simulink model "missile_model_3"  (R2022b)
settings: Solver=ode4  StartTime=0.0  StopTime=50  FixedStep=0.01  RelTol=1e-3
InitFcn:
  | clc, clear, close all
  | UAV_Data
  | Sim_Parameters
values from neighbouring files (symbols this model uses):
  Alt_Trim = 0    [Missile_Trim_Solution.mat]    (also in Trim_Main_missile.m = 4000; Trim_Solution_missile1.mat; Trim_Solution_missile2.mat; Trim_Solution_missile3.mat)
  D = 0.150    (= 0.15)    [UAV_Data.m]    (also in UAV_Data.mat)
  G_Turn = Turn_dot_Trim * Speed_Trim / UNIT_GRAV    [Trim_Main_missile.m]
  Gamma_Trim = 0.0 * UNIT_DEG2RAD    [Trim_Main_missile.m]
  Init_Cnstr1 = 0.0    (= 0)    [Trim_Main_missile.m]
  Init_Cnstr2 = 0.0    (= 0)    [Trim_Main_missile.m]
  Init_Cnstr3 = 0.0    (= 0)    [Trim_Main_missile.m]
  K_A = 0.0270    (= 0.027)    [UAV_Data.m]    (also in UAV_Data.mat)
  K_DC = 0.8443/10    (= 0.08443)    [UAV_Data.m]    (also in UAV_Data.mat = 0.8443)
  K_p = 0.01    [UAV_Data.m]    (also in UAV_Data.mat)
  K_phi = 20.0*2    (= 40)    [UAV_Data.m]    (also in UAV_Data.mat = 20)
  K_R = 0.0777    [UAV_Data.m]    (also in UAV_Data.mat)
  Mass = 30.0    (= 30)    [UAV_Data.m]    (also in UAV_Data.mat)
  Omega_i = -6.5208/5    (= -1.30416)    [UAV_Data.m]    (also in UAV_Data.mat = -6.5208)
  S = dat.S    [Assigment3_work.m]    (also in Missile_EoM.m; UAV_Data.m = 0.0176714586764; UAV_Data.mat = 0.0176714586764; verify_coeff.m)
  Speed_Trim = 102.088237307    [Missile_Trim_Solution.mat]    (also in Trim_Main_missile.m = 227.1878; Trim_Solution_missile1.mat = 102.0804; Trim_Solution_missile2.mat = 136.1072; Trim_Solution_missile3.mat = 204.1608)
  UNIT_GRAV = 9.81    [Sim_Parameters.m]
  Wn_Act = 25.0 * 2 * pi    (= 157.079632679)    [UAV_Data.m]    (also in UAV_Data.mat)
  Zeta_Act = 0.707    [UAV_Data.m]    (also in UAV_Data.mat)
libraries: aerolibconvert2 x3, aerolibasang x2, shared6dof x1, aerolibtransform2 x1, aerolibatmos2 x1
settings Model: Creator=Komsun  LastModifiedBy=Komsun

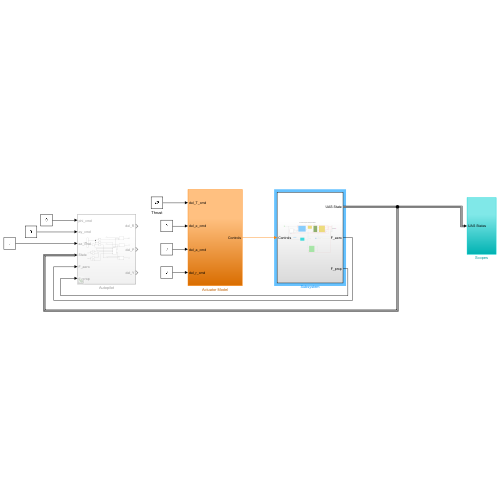
[thumbnail: Simulink's stored preview of the top-level diagram]
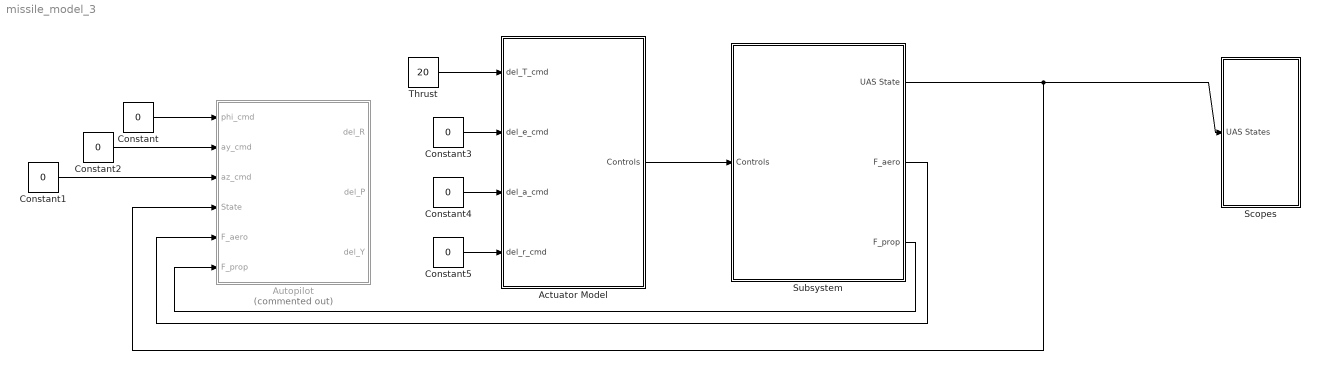
== system missile_model_3 ==
  Actuator Model : Subsystem
  Autopilot : Subsystem  Commented=on
  Constant{,1..5} (6 alike) : Constant  Value=0
  Scopes : Subsystem
  Subsystem : Subsystem
  Thrust : Constant  Value=20
  wires:
  Subsystem/1(UAS State) -> Autopilot/4(State), Scopes/1(UAS States)
  Constant/1 -> Autopilot/1(phi_cmd)
  Thrust/1 -> Actuator Model/1(del_T_cmd)
  Constant1/1 -> Autopilot/3(az_cmd)
  Actuator Model/1(Controls) -> Subsystem/1(Controls)
  Constant2/1 -> Autopilot/2(ay_cmd)
  Subsystem/2(F_aero) -> Autopilot/5(F_aero)
  Subsystem/3(F_prop) -> Autopilot/6(F_prop)
  Constant3/1 -> Actuator Model/2(del_e_cmd)
  Constant4/1 -> Actuator Model/3(del_a_cmd)
  Constant5/1 -> Actuator Model/4(del_r_cmd)

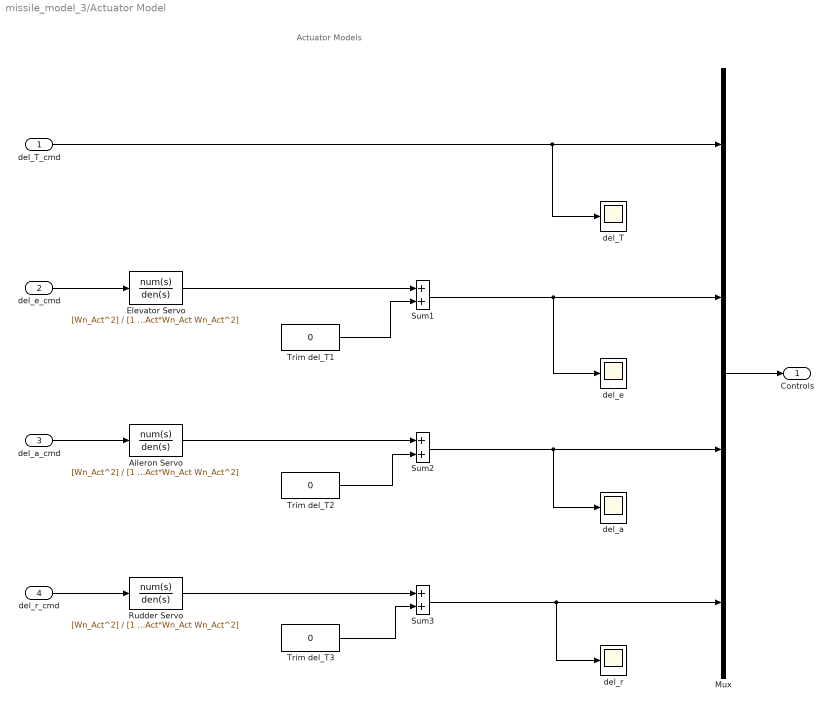
== system missile_model_3/Actuator Model ==
  note: Actuator Models
  del_T_cmd : Inport
  del_e_cmd : Inport  Port=2
  del_a_cmd : Inport  Port=3
  del_r_cmd : Inport  Port=4
  Aileron Servo : TransferFcn  Numerator=[Wn_Act^2]  Denominator=[1 2*Zeta_Act*Wn_Act Wn_Act^2]
  Elevator Servo : TransferFcn  Numerator=[Wn_Act^2]  Denominator=[1 2*Zeta_Act*Wn_Act Wn_Act^2]
  Mux : Mux
  Rudder Servo : TransferFcn  Numerator=[Wn_Act^2]  Denominator=[1 2*Zeta_Act*Wn_Act Wn_Act^2]
  Sum1 : Sum  SaturateOnIntegerOverflow=on
  Sum2 : Sum  SaturateOnIntegerOverflow=on
  Sum3 : Sum  SaturateOnIntegerOverflow=on
  Trim del_T1 : Constant  Value=0
  Trim del_T2 : Constant  Value=0
  Trim del_T3 : Constant  Value=0
  del_T : Scope
  del_a : Scope
  del_e : Scope
  del_r : Scope
  Controls : Outport
  wires:
  Mux/1 -> Controls/1
  del_T_cmd/1 -> del_T/1, Mux/1
  del_e_cmd/1 -> Elevator Servo/1
  Elevator Servo/1 -> Sum1/1
  Sum1/1 -> del_e/1, Mux/2
  Trim del_T1/1 -> Sum1/2
  Sum2/1 -> del_a/1, Mux/3
  Aileron Servo/1 -> Sum2/1
  Trim del_T2/1 -> Sum2/2
  del_a_cmd/1 -> Aileron Servo/1
  Sum3/1 -> del_r/1, Mux/4
  Trim del_T3/1 -> Sum3/2
  Rudder Servo/1 -> Sum3/1
  del_r_cmd/1 -> Rudder Servo/1

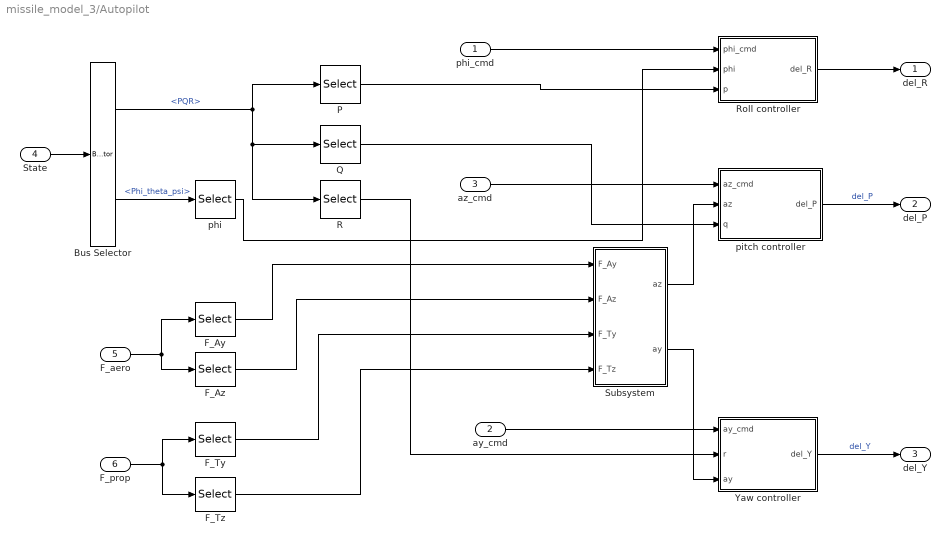
== system missile_model_3/Autopilot ==
  phi_cmd : Inport
  ay_cmd : Inport  Port=2
  az_cmd : Inport  Port=3
  State : Inport  Port=4
  F_aero : Inport  Port=5
  F_prop : Inport  Port=6
  Bus Selector : BusSelector  OutputSignals=PQR,Phi_theta_psi
  F_Ay : Selector  InputPortWidth=3  IndexOptions=Index vector (dialog)  Indices=[2]  OutputSizes=1
  F_Az : Selector  InputPortWidth=3  IndexOptions=Index vector (dialog)  Indices=[3]  OutputSizes=1
  F_Ty : Selector  InputPortWidth=3  IndexOptions=Index vector (dialog)  Indices=[2]  OutputSizes=1
  F_Tz : Selector  InputPortWidth=3  IndexOptions=Index vector (dialog)  Indices=[3]  OutputSizes=1
  P : Selector  InputPortWidth=3  IndexOptions=Index vector (dialog)  Indices=[1]  OutputSizes=1
  Q : Selector  InputPortWidth=3  IndexOptions=Index vector (dialog)  Indices=[2]  OutputSizes=1
  R : Selector  InputPortWidth=3  IndexOptions=Index vector (dialog)  Indices=[3]  OutputSizes=1
  Roll controller : Subsystem
  Subsystem : Subsystem
  Yaw controller : Subsystem
  phi : Selector  InputPortWidth=3  IndexOptions=Index vector (dialog)  Indices=[1]  OutputSizes=1
  pitch controller : Subsystem
  del_R : Outport
  del_P : Outport  Port=2
  del_Y : Outport  Port=3
  wires:
  pitch controller/1(del_P) -> del_P/1  "del_P"
  Yaw controller/1(del_Y) -> del_Y/1  "del_Y"
  phi_cmd/1 -> Roll controller/1(phi_cmd)
  Roll controller/1(del_R) -> del_R/1
  az_cmd/1 -> pitch controller/1(az_cmd)
  Subsystem/1(az) -> pitch controller/2(az)
  ay_cmd/1 -> Yaw controller/1(ay_cmd)
  Subsystem/2(ay) -> Yaw controller/3(ay)
  State/1 -> Bus Selector/1
  F_aero/1 -> F_Az/1, F_Ay/1
  F_Ay/1 -> Subsystem/1(F_Ay)
  F_Az/1 -> Subsystem/2(F_Az)
  F_prop/1 -> F_Ty/1, F_Tz/1
  F_Ty/1 -> Subsystem/3(F_Ty)
  F_Tz/1 -> Subsystem/4(F_Tz)
  Bus Selector/1 -> R/1, Q/1, P/1  "<PQR>"
  P/1 -> Roll controller/3(p)
  Q/1 -> pitch controller/3(q)
  R/1 -> Yaw controller/2(r)
  Bus Selector/2 -> phi/1  "<Phi_theta_psi>"
  phi/1 -> Roll controller/2(phi)

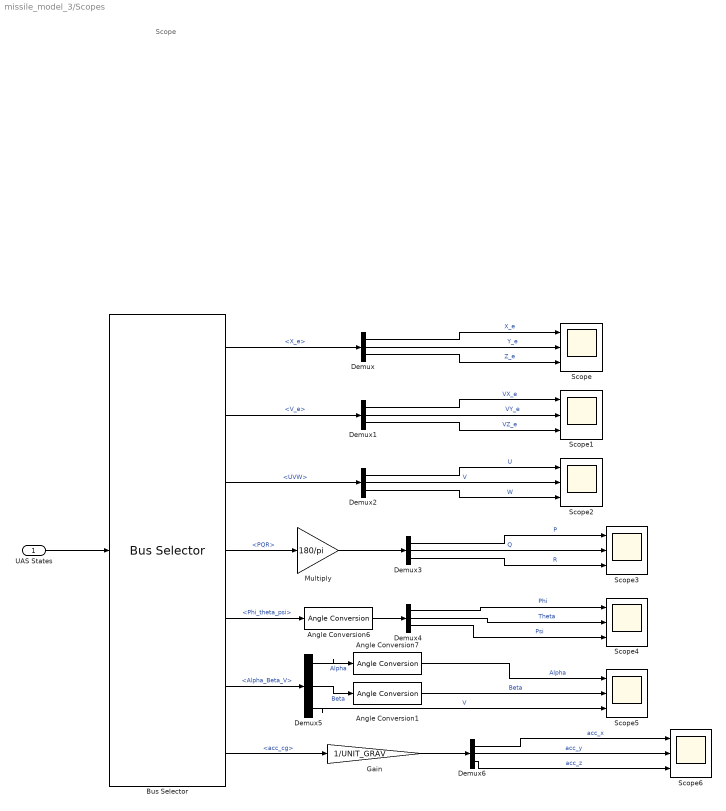
== system missile_model_3/Scopes ==
  note: Scope
  UAS States : Inport
  Angle Conversion1 : aerolibconvert2/Angle Conversion  IU=rad  OU=deg
  Angle Conversion6 : aerolibconvert2/Angle Conversion  IU=rad  OU=deg
  Angle Conversion7 : aerolibconvert2/Angle Conversion  IU=rad  OU=deg
  Bus Selector : BusSelector  OutputSignals=X_e,V_e,UVW,PQR,Phi_theta_psi,Alpha_Beta_V,acc_cg
  Demux{,1..6} (7 alike) : Demux  Outputs=3
  Gain : Gain  Gain=1/UNIT_GRAV
  Multiply : Gain  Gain=180/pi
  Scope{,1..6} (7 alike) : Scope  NumInputPorts=3
  wires:
  UAS States/1 -> Bus Selector/1
  Demux/1 -> Scope/1  "X_e"
  Demux/2 -> Scope/2  "Y_e"
  Demux/3 -> Scope/3  "Z_e"
  Bus Selector/4 -> Multiply/1  "<PQR>"
  Bus Selector/5 -> Angle Conversion6/1  "<Phi_theta_psi>"
  Bus Selector/6 -> Demux5/1  "<Alpha_Beta_V>"
  Bus Selector/7 -> Gain/1  "<acc_cg>"
  Bus Selector/1 -> Demux/1  "<X_e>"
  Demux1/3 -> Scope1/3  "VZ_e"
  Demux1/1 -> Scope1/1  "VX_e"
  Demux1/2 -> Scope1/2  "VY_e"
  Bus Selector/2 -> Demux1/1  "<V_e>"
  Bus Selector/3 -> Demux2/1  "<UVW>"
  Demux2/2 -> Scope2/2  "V"
  Demux2/1 -> Scope2/1  "U"
  Demux2/3 -> Scope2/3  "W"
  Demux3/3 -> Scope3/3  "R"
  Demux3/1 -> Scope3/1  "P"
  Demux3/2 -> Scope3/2  "Q"
  Multiply/1 -> Demux3/1
  Angle Conversion6/1 -> Demux4/1
  Demux4/2 -> Scope4/2  "Theta"
  Demux4/1 -> Scope4/1  "Phi"
  Demux4/3 -> Scope4/3  "Psi"
  Demux5/2 -> Angle Conversion1/1  "Beta"
  Demux5/3 -> Scope5/3  "V"
  Demux5/1 -> Angle Conversion7/1  "Alpha"
  Demux6/1 -> Scope6/1  "acc_x"
  Demux6/2 -> Scope6/2  "acc_y"
  Gain/1 -> Demux6/1
  Demux6/3 -> Scope6/3  "acc_z"
  Angle Conversion7/1 -> Scope5/1  "Alpha"
  Angle Conversion1/1 -> Scope5/2  "Beta"

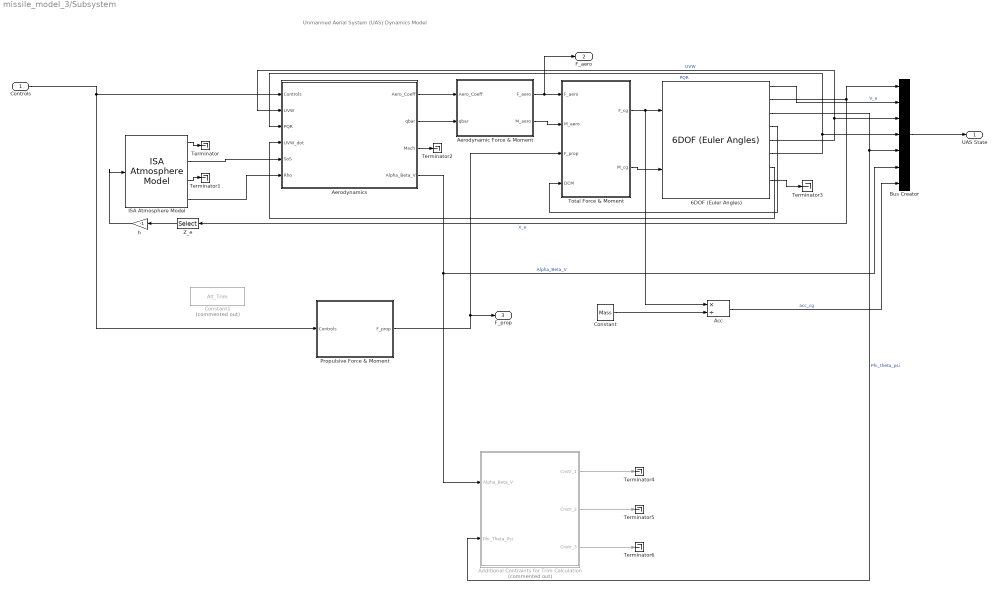
== system missile_model_3/Subsystem ==
  note: Unmanned Aerial System (UAS) Dynamics Model
  Controls : Inport
  6DOF (Euler Angles) : shared6dof/6DOF (Euler Angles)  units=Metric (MKS)  mtype=Fixed  rep=Euler Angles  xme_0=Init_Pos  Vm_0=Init_Vel  eul_0=[0 0 0]  pm_0=[0 0 0]  mass_0=30  mass_e=0.5  mass_f=2.0  inertia=I_TENSOR  inertia_e=eye(3)  inertia_f=2*eye(3)  k_quat=1.0  vre_flag=on  abi_flag=on  aMode=0  xme_statename=''  Vm_statename=''  eul_statename=''  quat_statename=''  pm_statename=''  mass_statename=''
  Acc : Product  Inputs=*/  RndMeth=Zero
  Additional Contraints for Trim Calculation : Subsystem  Commented=on
  Aerodynamic Force & Moment : Subsystem
  Aerodynamics : Subsystem
  Bus Creator : BusCreator  Inputs=7
  Constant : Constant  Value=Mass
  Constant1 : Constant  Commented=on  Value=Alt_Trim
  ISA Atmosphere Model : aerolibatmos2/ISA Atmosphere Model  custom=off  g=9.80665  gamma=1.4  R=287.0531  L=0.0065  h_trop=11000  h_strat=20000  rho0=1.225  P0=101325  T0=288.15  h0=0
  Propulsive Force & Moment : Subsystem
  Terminator{,1..6} (7 alike) : Terminator
  Total Force & Moment : Subsystem
  Z_e : Selector  InputPortWidth=3  IndexOptions=Index vector (dialog)  Indices=[3]  OutputSizes=1
  h : Gain  Gain=-1
  UAS State : Outport
  F_aero : Outport  Port=2
  F_prop : Outport  Port=3
  wires:
  6DOF (Euler Angles)/3 -> Bus Creator/5, Additional Contraints for Trim Calculation/2(Phi_Theta_Psi)  "Phi_theta_psi"
  Additional Contraints for Trim Calculation/2(Cnstr_2) -> Terminator5/1
  Aerodynamics/4(Alpha_Beta_V) -> Bus Creator/6, Additional Contraints for Trim Calculation/1(Alpha_Beta_V)  "Alpha_Beta_V"
  Propulsive Force & Moment/1(F_prop) -> F_prop/1, Total Force & Moment/3(F_prop)
  Additional Contraints for Trim Calculation/1(Cnstr_1) -> Terminator4/1
  h/1 -> ISA Atmosphere Model/1
  ISA Atmosphere Model/2 -> Aerodynamics/5(SoS)
  6DOF (Euler Angles)/7 -> Aerodynamics/4("UVW_dot ")
  Z_e/1 -> h/1
  Aerodynamics/1(Aero_Coeff) -> Aerodynamic Force & Moment/1(Aero_Coeff)
  Aerodynamic Force & Moment/1(F_aero) -> F_aero/1, Total Force & Moment/1(F_aero)
  ISA Atmosphere Model/1 -> Terminator/1
  ISA Atmosphere Model/3 -> Terminator1/1
  Acc/1 -> Bus Creator/7  "acc_cg"
  6DOF (Euler Angles)/5 -> Bus Creator/3, Aerodynamics/2(UVW)  "UVW"
  Controls/1 -> Propulsive Force & Moment/1(Controls), Aerodynamics/1(Controls)
  Aerodynamic Force & Moment/2(M_aero) -> Total Force & Moment/2(M_aero)
  Aerodynamics/3(Mach) -> Terminator2/1
  Aerodynamics/2(qbar) -> Aerodynamic Force & Moment/2(qbar)
  Additional Contraints for Trim Calculation/3(Cnstr_3) -> Terminator6/1
  Total Force & Moment/1(F_cg) -> Acc/1, 6DOF (Euler Angles)/1
  Total Force & Moment/2(M_cg) -> 6DOF (Euler Angles)/2
  6DOF (Euler Angles)/1 -> Bus Creator/2  "V_e"
  Constant/1 -> Acc/2
  ISA Atmosphere Model/4 -> Aerodynamics/6(Rho)
  6DOF (Euler Angles)/6 -> Bus Creator/4, Aerodynamics/3(PQR)  "PQR"
  6DOF (Euler Angles)/2 -> Z_e/1, Bus Creator/1  "X_e"
  6DOF (Euler Angles)/4 -> Total Force & Moment/4(DCM)
  Bus Creator/1 -> UAS State/1
  6DOF (Euler Angles)/8 -> Terminator3/1

== system missile_model_3/Autopilot/Roll controller ==
  phi_cmd : Inport
  phi : Inport  Port=2
  p : Inport  Port=3
  K_p : Gain  Gain=K_p
  K_phi : Gain  Gain=K_phi
  Sum : Sum  Inputs=|+-
  Sum1 : Sum  Inputs=|+-
  del_R : Outport
  wires:
  p/1 -> Sum/2
  K_p/1 -> del_R/1  "del_R"
  Sum/1 -> K_phi/1
  phi/1 -> Sum1/2
  Sum1/1 -> K_p/1
  K_phi/1 -> Sum1/1
  phi_cmd/1 -> Sum/1

== system missile_model_3/Autopilot/Subsystem ==
  F_Ay : Inport
  F_Az : Inport  Port=2
  F_Ty : Inport  Port=3
  F_Tz : Inport  Port=4
  Divide : Product  Inputs=*/
  Divide1 : Product  Inputs=*/
  Mass : Constant  Value=Mass
  Sum : Sum  Inputs=|++
  Sum1 : Sum  Inputs=|++
  az : Outport
  ay : Outport  Port=2
  wires:
  F_Ay/1 -> Sum1/1  "F_Ay"
  Mass/1 -> Divide1/2, Divide/2
  Sum/1 -> Divide/1
  F_Ty/1 -> Sum1/2  "F_Ty"
  Sum1/1 -> Divide1/1
  F_Az/1 -> Sum/1  "F_Az"
  Divide/1 -> az/1
  F_Tz/1 -> Sum/2  "F_Tz"
  Divide1/1 -> ay/1

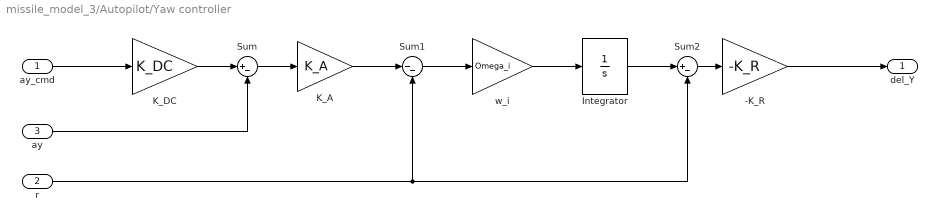
== system missile_model_3/Autopilot/Yaw controller ==
  ay_cmd : Inport
  r : Inport  Port=2
  ay : Inport  Port=3
  -K_R : Gain  Gain=-K_R
  Integrator : Integrator
  K_A : Gain  Gain=K_A
  K_DC : Gain  Gain=K_DC
  Sum : Sum  Inputs=|+-
  Sum1 : Sum  Inputs=|--
  Sum2 : Sum  Inputs=|+-
  w_i : Gain  Gain=Omega_i
  del_Y : Outport
  wires:
  ay_cmd/1 -> K_DC/1
  r/1 -> Sum2/2, Sum1/2
  K_DC/1 -> Sum/1
  ay/1 -> Sum/2
  Sum/1 -> K_A/1
  K_A/1 -> Sum1/1
  Sum1/1 -> w_i/1
  w_i/1 -> Integrator/1
  Integrator/1 -> Sum2/1
  Sum2/1 -> -K_R/1
  -K_R/1 -> del_Y/1

== system missile_model_3/Autopilot/pitch controller ==
  az_cmd : Inport
  az : Inport  Port=2
  q : Inport  Port=3
  Integrator : Integrator
  K_A : Gain  Gain=K_A
  K_DC : Gain  Gain=K_DC
  K_R : Gain  Gain=K_R
  Sum : Sum  Inputs=|+-
  Sum1 : Sum  Inputs=|-+
  Sum2 : Sum  Inputs=|++
  w_i : Gain  Gain=Omega_i
  del_P : Outport
  wires:
  az_cmd/1 -> K_DC/1
  K_DC/1 -> Sum/1
  az/1 -> Sum/2
  Sum/1 -> K_A/1
  K_A/1 -> Sum1/1
  q/1 -> Sum2/2, Sum1/2
  Sum1/1 -> w_i/1
  w_i/1 -> Integrator/1
  Integrator/1 -> Sum2/1
  Sum2/1 -> K_R/1
  K_R/1 -> del_P/1

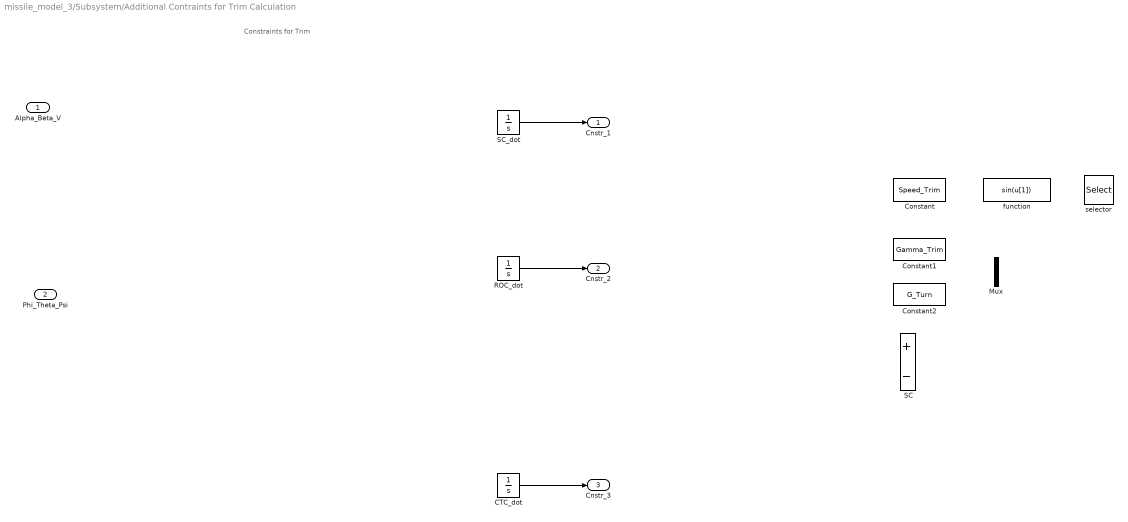
== system missile_model_3/Subsystem/Additional Contraints for Trim Calculation ==
  note: Constraints for Trim
  Alpha_Beta_V : Inport  PortDimensions=3
  Phi_Theta_Psi : Inport  Port=2  PortDimensions=3
  CTC_dot : Integrator  InitialCondition=Init_Cnstr3
  Constant : Constant  Value=Speed_Trim
  Constant1 : Constant  Value=Gamma_Trim
  Constant2 : Constant  Value=G_Turn
  Mux : Mux  Inputs=2
  ROC_dot : Integrator  InitialCondition=Init_Cnstr2
  SC : Sum  Inputs=+-
  SC_dot : Integrator  InitialCondition=Init_Cnstr1
  function : Fcn
  selector : Selector  InputPortWidth=3  IndexOptions=Index vector (dialog)  Indices=[3]  OutputSizes=1
  Cnstr_1 : Outport
  Cnstr_2 : Outport  Port=2
  Cnstr_3 : Outport  Port=3
  wires:
  SC_dot/1 -> Cnstr_1/1
  ROC_dot/1 -> Cnstr_2/1
  CTC_dot/1 -> Cnstr_3/1

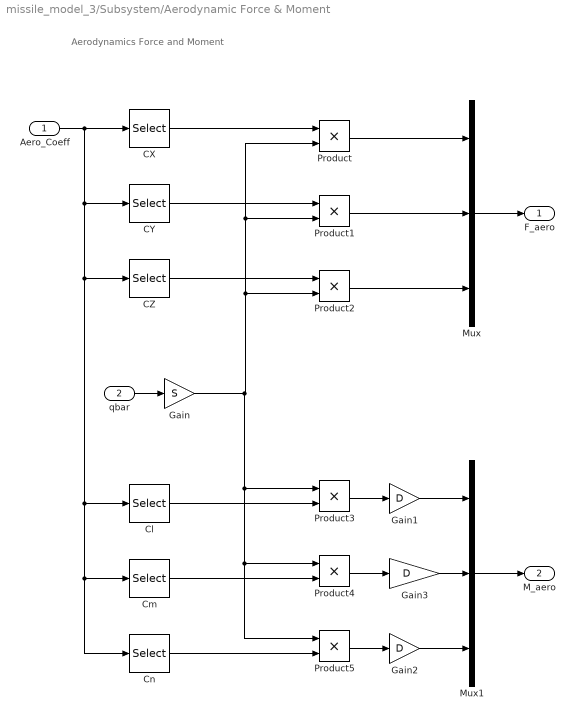
== system missile_model_3/Subsystem/Aerodynamic Force & Moment ==
  note: Aerodynamics Force and Moment
  Aero_Coeff : Inport
  qbar : Inport  Port=2
  CX : Selector  InputPortWidth=6  IndexOptions=Index vector (dialog)  Indices=[1]  OutputSizes=1
  CY : Selector  InputPortWidth=6  IndexOptions=Index vector (dialog)  Indices=[2]  OutputSizes=1
  CZ : Selector  InputPortWidth=6  IndexOptions=Index vector (dialog)  Indices=[3]  OutputSizes=1
  Cl : Selector  InputPortWidth=6  IndexOptions=Index vector (dialog)  Indices=[4]  OutputSizes=1
  Cm : Selector  InputPortWidth=6  IndexOptions=Index vector (dialog)  Indices=[5]  OutputSizes=1
  Cn : Selector  InputPortWidth=6  IndexOptions=Index vector (dialog)  Indices=[6]  OutputSizes=1
  Gain : Gain  Gain=S
  Gain1 : Gain  Gain=D
  Gain2 : Gain  Gain=D
  Gain3 : Gain  Gain=D
  Mux : Mux  Inputs=3
  Mux1 : Mux  Inputs=3
  Product{,1..5} (6 alike) : Product
  F_aero : Outport
  M_aero : Outport  Port=2
  wires:
  Aero_Coeff/1 -> Cl/1, Cn/1, Cm/1, CZ/1, CY/1, CX/1
  qbar/1 -> Gain/1
  CX/1 -> Product/1
  Gain/1 -> Product5/1, Product4/1, Product3/1, Product2/2, Product1/2, Product/2
  CY/1 -> Product1/1
  CZ/1 -> Product2/1
  Product/1 -> Mux/1
  Product1/1 -> Mux/2
  Product2/1 -> Mux/3
  Mux/1 -> F_aero/1
  Cl/1 -> Product3/2
  Cm/1 -> Product4/2
  Cn/1 -> Product5/2
  Product3/1 -> Gain1/1
  Product4/1 -> Gain3/1
  Product5/1 -> Gain2/1
  Mux1/1 -> M_aero/1
  Gain1/1 -> Mux1/1
  Gain2/1 -> Mux1/3
  Gain3/1 -> Mux1/2

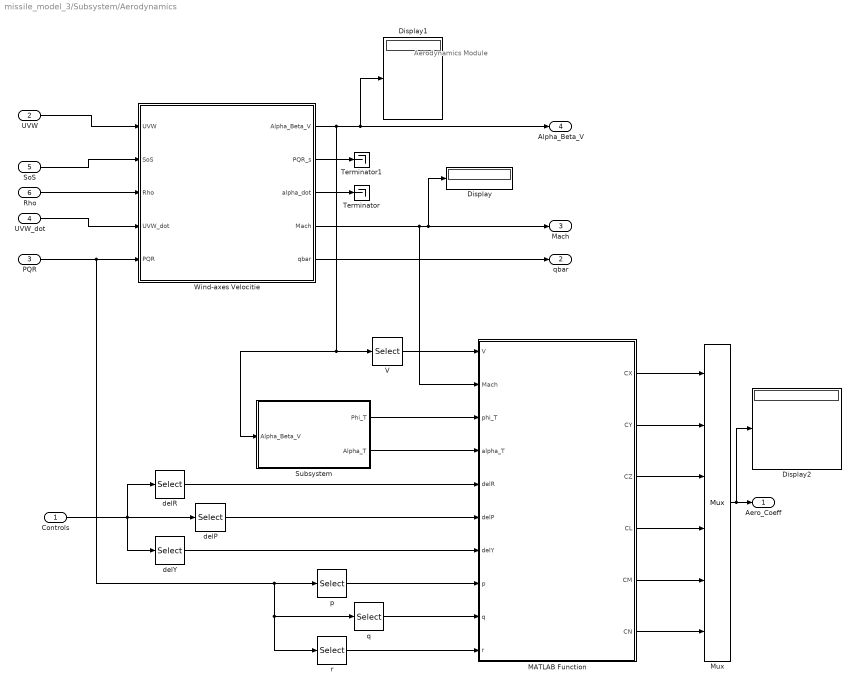
== system missile_model_3/Subsystem/Aerodynamics ==
  note: Aerodynamics Module
  Controls : Inport
  UVW : Inport  Port=2
  PQR : Inport  Port=3
  "UVW_dot " : Inport  Port=4
  SoS : Inport  Port=5
  Rho : Inport  Port=6
  Display : Display
  Display1 : Display
  Display2 : Display
  MATLAB Function : MATLAB Function  TreatAsAtomicUnit=on
  Mux : Mux  Inputs=6
  Subsystem : Subsystem
  Terminator : Terminator
  Terminator1 : Terminator
  V : Selector  InputPortWidth=3  IndexOptions=Index vector (dialog)  Indices=[3]  OutputSizes=1
  Wind-axes Velocitie : Subsystem
  delP : Selector  InputPortWidth=4  IndexOptions=Index vector (dialog)  Indices=[3]  OutputSizes=1
  delR : Selector  InputPortWidth=4  IndexOptions=Index vector (dialog)  Indices=[2]  OutputSizes=1
  delY : Selector  InputPortWidth=4  IndexOptions=Index vector (dialog)  Indices=[4]  OutputSizes=1
  p : Selector  InputPortWidth=3  IndexOptions=Index vector (dialog)  Indices=[1]  OutputSizes=1
  q : Selector  InputPortWidth=3  IndexOptions=Index vector (dialog)  Indices=[2]  OutputSizes=1
  r : Selector  InputPortWidth=3  IndexOptions=Index vector (dialog)  Indices=[3]  OutputSizes=1
  Aero_Coeff : Outport
  qbar : Outport  Port=2
  Mach : Outport  Port=3
  Alpha_Beta_V : Outport  Port=4
  wires:
  Wind-axes Velocitie/1(Alpha_Beta_V) -> Subsystem/1(Alpha_Beta_V), V/1, Display1/1, Alpha_Beta_V/1
  UVW/1 -> Wind-axes Velocitie/1(UVW)
  Mux/1 -> Display2/1, Aero_Coeff/1
  Wind-axes Velocitie/4(Mach) -> MATLAB Function/2(Mach), Mach/1, Display/1
  Wind-axes Velocitie/5(qbar) -> qbar/1
  SoS/1 -> Wind-axes Velocitie/2(SoS)
  Rho/1 -> Wind-axes Velocitie/3(Rho)
  "UVW_dot "/1 -> Wind-axes Velocitie/4(UVW_dot)
  PQR/1 -> r/1, q/1, p/1, Wind-axes Velocitie/5(PQR)
  Wind-axes Velocitie/3(alpha_dot) -> Terminator/1
  Wind-axes Velocitie/2(PQR_s) -> Terminator1/1
  Subsystem/2(Alpha_T) -> MATLAB Function/4(alpha_T)
  V/1 -> MATLAB Function/1(V)
  Subsystem/1(Phi_T) -> MATLAB Function/3(phi_T)
  Controls/1 -> delY/1, delR/1, delP/1
  delR/1 -> MATLAB Function/5(delR)
  delP/1 -> MATLAB Function/6(delP)
  delY/1 -> MATLAB Function/7(delY)
  p/1 -> MATLAB Function/8(p)
  q/1 -> MATLAB Function/9(q)
  r/1 -> MATLAB Function/10(r)
  MATLAB Function/1(CX) -> Mux/1
  MATLAB Function/2(CY) -> Mux/2
  MATLAB Function/3(CZ) -> Mux/3
  MATLAB Function/4(CL) -> Mux/4
  MATLAB Function/5(CM) -> Mux/5
  MATLAB Function/6(CN) -> Mux/6

== system missile_model_3/Subsystem/Propulsive Force & Moment ==
  note: Propulsive Force and Moment
  Controls : Inport
  Constant : Constant  Value=0
  Mux : Mux  Inputs=3
  Thrust : Selector  InputPortWidth=4  IndexOptions=Index vector (dialog)  Indices=[1]  OutputSizes=1
  F_prop : Outport
  wires:
  Constant/1 -> Mux/3, Mux/2
  Controls/1 -> Thrust/1
  Thrust/1 -> Mux/1
  Mux/1 -> F_prop/1

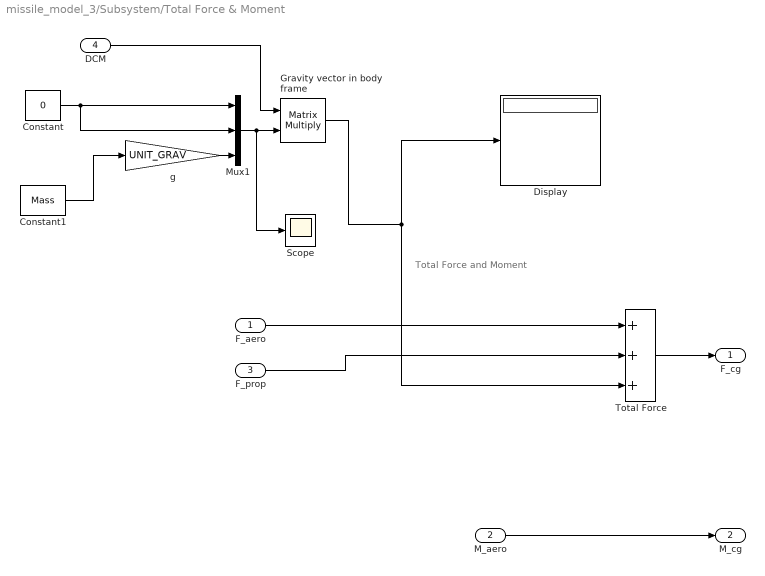
== system missile_model_3/Subsystem/Total Force & Moment ==
  note: Total Force and Moment
  F_aero : Inport  PortDimensions=3
  M_aero : Inport  Port=2  PortDimensions=3
  F_prop : Inport  Port=3  PortDimensions=3
  DCM : Inport  Port=4
  Constant : Constant  Value=0
  Constant1 : Constant  Value=Mass
  Display : Display
  "Gravity vector in body frame " : Product  Multiplication=Matrix(*)  InputSameDT=on  SaturateOnIntegerOverflow=on  OutDataTypeStr=Inherit: Same as first input
  Mux1 : Mux  Inputs=3
  Scope : Scope
  Total Force : Sum  Inputs=+++  InputSameDT=on  SaturateOnIntegerOverflow=on  OutDataTypeStr=Inherit: Same as first input
  g : Gain  Gain=UNIT_GRAV
  F_cg : Outport
  M_cg : Outport  Port=2
  wires:
  Total Force/1 -> F_cg/1
  F_aero/1 -> Total Force/1
  F_prop/1 -> Total Force/2
  M_aero/1 -> M_cg/1
  Mux1/1 -> Scope/1, "Gravity vector in body frame "/2
  "Gravity vector in body frame "/1 -> Total Force/3, Display/1
  Constant1/1 -> g/1
  Constant/1 -> Mux1/2, Mux1/1
  g/1 -> Mux1/3
  DCM/1 -> "Gravity vector in body frame "/1

== system missile_model_3/Subsystem/Aerodynamics/Subsystem ==
  Alpha_Beta_V : Inport
  Acos : Trigonometry  Operator=acos
  Atan2 : Trigonometry  Operator=atan2
  Beta : Selector  InputPortWidth=3  IndexOptions=Index vector (dialog)  Indices=[2]  OutputSizes=1
  Cos1 : Trigonometry  Operator=cos
  Cos2 : Trigonometry  Operator=cos
  Product : Product
  Sin : Trigonometry
  Tan : Trigonometry  Operator=tan
  alpha : Selector  InputPortWidth=3  IndexOptions=Index vector (dialog)  Indices=[1]  OutputSizes=1
  Phi_T : Outport
  Alpha_T : Outport  Port=2
  wires:
  Alpha_Beta_V/1 -> alpha/1, Beta/1
  Beta/1 -> Tan/1, Cos2/1
  Tan/1 -> Atan2/1
  Sin/1 -> Atan2/2
  Atan2/1 -> Phi_T/1
  alpha/1 -> Cos1/1, Sin/1
  Cos1/1 -> Product/1
  Cos2/1 -> Product/2
  Product/1 -> Acos/1
  Acos/1 -> Alpha_T/1

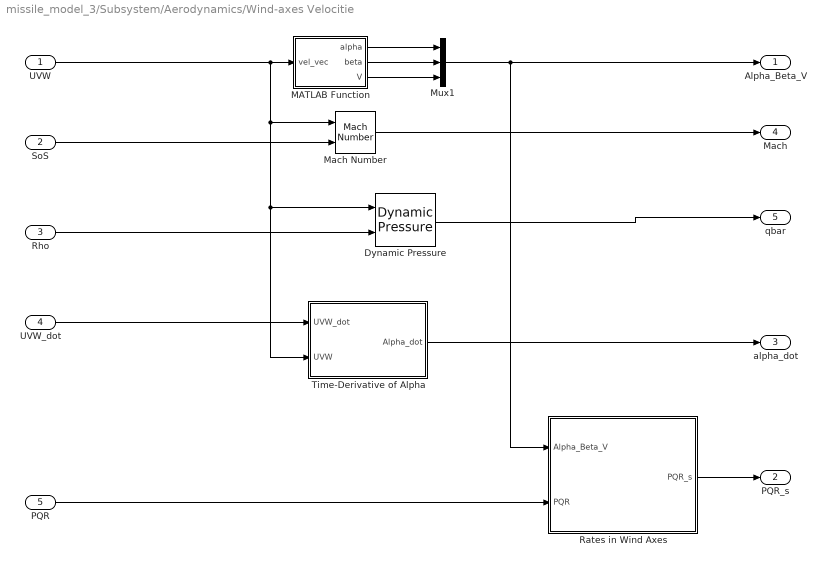
== system missile_model_3/Subsystem/Aerodynamics/Wind-axes Velocitie ==
  UVW : Inport
  SoS : Inport  Port=2
  Rho : Inport  Port=3
  UVW_dot : Inport  Port=4
  PQR : Inport  Port=5
  Dynamic Pressure : aerolibasang/Dynamic Pressure
  MATLAB Function : MATLAB Function  TreatAsAtomicUnit=on
  Mach Number : aerolibasang/Mach Number
  Mux1 : Mux  Inputs=3
  Rates in Wind Axes : Subsystem
  Time-Derivative of Alpha : Subsystem
  Alpha_Beta_V : Outport
  PQR_s : Outport  Port=2
  alpha_dot : Outport  Port=3
  Mach : Outport  Port=4
  qbar : Outport  Port=5
  wires:
  UVW_dot/1 -> Time-Derivative of Alpha/1(UVW_dot)
  Time-Derivative of Alpha/1(Alpha_dot) -> alpha_dot/1
  Dynamic Pressure/1 -> qbar/1
  Rho/1 -> Dynamic Pressure/2
  SoS/1 -> Mach Number/2
  Mach Number/1 -> Mach/1
  Mux1/1 -> Rates in Wind Axes/1(Alpha_Beta_V), Alpha_Beta_V/1
  UVW/1 -> Mach Number/1, Time-Derivative of Alpha/2(UVW), Dynamic Pressure/1, MATLAB Function/1(vel_vec)
  MATLAB Function/1(alpha) -> Mux1/1
  MATLAB Function/2(beta) -> Mux1/2
  MATLAB Function/3(V) -> Mux1/3
  Rates in Wind Axes/1(PQR_s) -> PQR_s/1
  PQR/1 -> Rates in Wind Axes/2(PQR)

== system missile_model_3/Subsystem/Aerodynamics/Wind-axes Velocitie/Rates in Wind Axes ==
  note: Rates in Wind Axes
  Alpha_Beta_V : Inport
  PQR : Inport  Port=2
  Alpha : Selector  InputPortWidth=3  IndexOptions=Index vector (dialog)  Indices=[1]  OutputSizes=1
  Beta_Ref : Constant  Value=0
  Direction Cosine Matrix Body to Wind : aerolibtransform2/Direction Cosine Matrix Body to Wind
  Mux : Mux  Inputs=2
  transform to body axes : Product  Inputs=**  Multiplication=Matrix(*)  InputSameDT=on  SaturateOnIntegerOverflow=on  OutDataTypeStr=Inherit: Same as first input
  PQR_s : Outport
  wires:
  Alpha_Beta_V/1 -> Alpha/1
  Alpha/1 -> Mux/1
  Direction Cosine Matrix Body to Wind/1 -> transform to body axes/1  "cB_W"
  PQR/1 -> transform to body axes/2
  transform to body axes/1 -> PQR_s/1
  Mux/1 -> Direction Cosine Matrix Body to Wind/1
  Beta_Ref/1 -> Mux/2

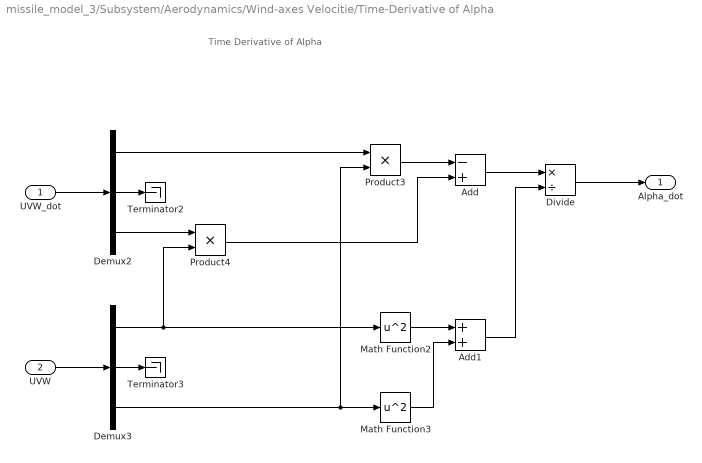
== system missile_model_3/Subsystem/Aerodynamics/Wind-axes Velocitie/Time-Derivative of Alpha ==
  note: Time Derivative of Alpha
  UVW_dot : Inport
  UVW : Inport  Port=2
  Add : Sum  Inputs=-+
  Add1 : Sum
  Demux2 : Demux  Outputs=3
  Demux3 : Demux  Outputs=3
  Divide : Product  Inputs=*/
  Math Function2 : Math  Operator=square  SignedPower=on
  Math Function3 : Math  Operator=square  SignedPower=on
  Product3 : Product
  Product4 : Product
  Terminator2 : Terminator
  Terminator3 : Terminator
  Alpha_dot : Outport
  wires:
  UVW_dot/1 -> Demux2/1
  Demux2/2 -> Terminator2/1
  Demux2/1 -> Product3/1
  UVW/1 -> Demux3/1
  Demux3/2 -> Terminator3/1
  Demux3/3 -> Math Function3/1, Product3/2
  Demux2/3 -> Product4/1
  Demux3/1 -> Math Function2/1, Product4/2
  Product4/1 -> Add/2
  Product3/1 -> Add/1
  Add/1 -> Divide/1
  Math Function2/1 -> Add1/1
  Math Function3/1 -> Add1/2
  Add1/1 -> Divide/2
  Divide/1 -> Alpha_dot/1

== matlab function missile_model_3/Subsystem/Aerodynamics/Wind-axes Velocitie/MATLAB Function ==
  data: vel_vec input; alpha output; beta output; V output
function [alpha, beta, V] = calc_abv(vel_vec)

u = vel_vec(1);
v = vel_vec(2);
w = vel_vec(3);

V = norm([u v w]);          % [m/s] UAV total Speed
% V = sqrt(u^2 + v^2 + w^2);
alpha = atan2(w,u);          % [rad] angle of attack
beta  = asin(v/V);          % [rad] sideslip angles

end

== matlab function missile_model_3/Subsystem/Aerodynamics/MATLAB Function ==
  data: V input; Mach input; CX output; phi_T input; alpha_T input; delR input; delP input; delY input; CY output; CZ output; CL output; CM output; CN output; p input; q input; r input
function [CX, CY, CZ, CL, CM, CN] = AeroCoef(V, Mach,phi_T, alpha_T, delR, delP, delY, p, q, r)

dat = load('UAV_Data.mat');
% dat.Tbl_ALPHAT = dat.Tbl_ALPHAT * pi/180;    % convert to rad
% alpha_T = alpha_T *180/pi;            % convert to degree

del_eff = (abs(delP) + abs(delY))/2;


B2A = rot1(-phi_T);                            % Body-to-Aeroballistics

delARPY = B2A *[delR; delP; delY];
delR_A = delARPY(1);
delP_A = delARPY(2);
delY_A = delARPY(3);

pqrA = B2A * [p; q; r];
pA = pqrA(1);
qA = pqrA(2);
rA = pqrA(3);
method = 'spline'; % 'spline', 'nearest'

CX_a = interp1(dat.Tbl_MACH, dat.Tbl_CX_0, Mach, method) + interp1(dat.Tbl_MACH, dat.Tbl_CX_ALPHAT, Mach, method)*alpha_T...
     + interp1(dat.Tbl_MACH, dat.Tbl_CX_DEL_EFF, Mach, method)*(del_eff)^2;

CY_a = interp2(dat.Tbl_ALPHAT, dat.Tbl_MACH, dat.Tbl_CY_PHIT, alpha_T, Mach, method)*sin(4*phi_T)...
     + interp1(dat.Tbl_MACH, dat.Tbl_CY_DEL_Y, Mach, method)*delY_A;

CZ_a = interp2(dat.Tbl_ALPHAT, dat.Tbl_MACH, dat.Tbl_CZ_0, alpha_T, Mach, method)...
     + interp2(dat.Tbl_ALPHAT, dat.Tbl_MACH, dat.Tbl_CZ_PHIT, alpha_T, Mach, method)*(sin(2*phi_T))^2 ...
     + interp1(dat.Tbl_MACH, dat.Tbl_CZ_DEL_P, Mach, method)*delP_A;

CL_a = interp1(dat.Tbl_MACH, dat.Tbl_CL_ALPHAT, Mach, method)*(alpha_T^2)*sin(4*phi_T) ...
     + interp1(dat.Tbl_MACH, dat.Tbl_CL_P, Mach, method)*(dat.D/(2*V))*pA ...
     + interp1(dat.Tbl_MACH, dat.Tbl_CL_DEL_R, Mach, method)*delR_A;

CM_a = interp2(dat.Tbl_ALPHAT, dat.Tbl_MACH, dat.Tbl_CM_0, alpha_T, Mach, method) ...
     + interp2(dat.Tbl_ALPHAT, dat.Tbl_MACH, dat.Tbl_CM_PHIT, alpha_T, Mach, method)*(sin(2*phi_T))^2 ...
     + interp1(dat.Tbl_MACH, dat.Tbl_CM_Q, Mach, method)*(dat.D/(2*V))*qA ...
     + interp1(dat.Tbl_MACH, dat.Tbl_CM_DEL_P, Mach, method)*delP_A ...
     - CZ_a*(dat.XCG - dat.XREF)/dat.D;

CN_a = interp2(dat.Tbl_ALPHAT, dat.Tbl_MACH, dat.Tbl_CN_PHIT, alpha_T, Mach, method)*sin(4*phi_T)...
     + interp1(dat.Tbl_MACH, dat.Tbl_CN_R, Mach, method)*(dat.D/(2*V))*rA ...
     + interp1(dat.Tbl_MACH, dat.Tbl_CN_DEL_Y, Mach, method)*delY_A ...
     + CY_a*(dat.XCG - dat.XREF)/dat.D;

%% Aerodynamics Coefficients in body coordinate
CXYZ = B2A.' * [CX_a; CY_a; CZ_a];
CX = CXYZ(1);
CY = CXYZ(2);
CZ = CXYZ(3);

CLMN = B2A.' * [CL_a; CM_a; CN_a];
CL = CLMN(1);
CM = CLMN(2);
CN = CLMN(3);

function out = rot1(x)
    out = [1 0 0; 0 cos(x) sin(x); 0 -sin(x) cos(x)];
end

end
